simulink model "NPC_threelevel_PI_Controller"  (R2024a)
settings: Solver=ode4  StartTime=0.0  StopTime=0.1  FixedStep=1e-6  MaxStep=1e-4  RelTol=1e-3
InitFcn:
  | v=3000
  | r=0.000001
  | c=1000e-6
  | l=314
  | i=1000
  | r1=1000
  | t=1/3000
  | ma=2
  | f=2*pi*50
  | p1=(2*pi)/3
  | p2=-(2*pi)/3
libraries: spsIGBTDiodeLib x12, spsSeriesRLCBranchLib x12, spsVoltageMeasurementLib x12, simulink x6, spsDiodeLib x6, slpidlib x3, spsRMSLib x3, spsCurrentMeasurementLib x3, spsDCVoltageSourceLib x1, sps_lib x1
settings Model: Creator=dell  LastModifiedBy=prath
settings SolverCC: AlgebraicLoopSolver=TrustRegion
settings DataIOCC: ReturnWorkspaceOutputs=off
settings DebuggingCC: UnconnectedInputMsg=warning  UnconnectedOutputMsg=warning  UnconnectedLineMsg=warning  ArithmeticOperatorsInVariantConditions=warning
settings ModelReferenceCC: EnableRefExpFcnMdlSchedulingChecks=on
settings SFSimCC: SimUseLocalCustomCode=off  CustomCodeUndefinedFunction=UseInterfaceOnly
settings RTWCC: RTWUseLocalCustomCode=off  GPUComputeCapability=3.5
settings CodeAppCC: StateflowObjectComments=on
settings SimscapeCC: SimscapeNormalizeSystem=off

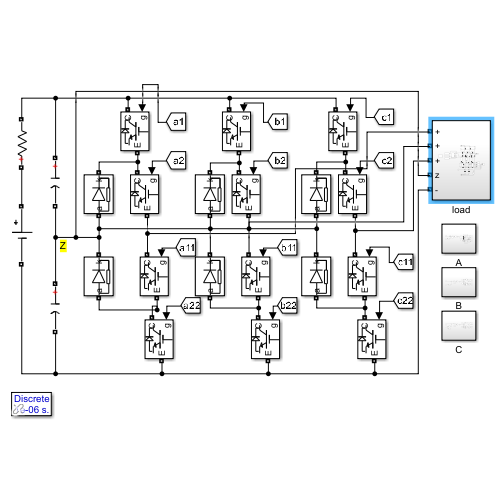
[thumbnail: Simulink's stored preview of the top-level diagram]
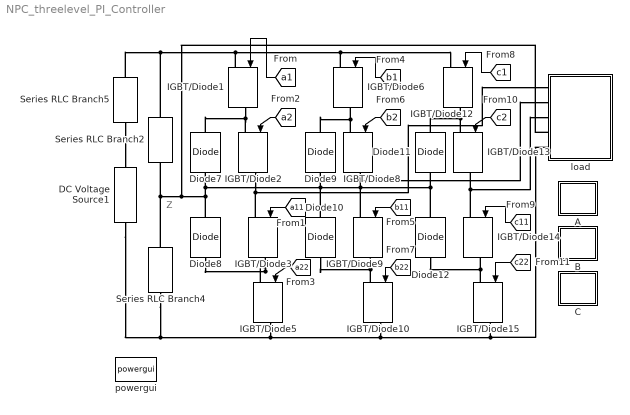
== system NPC_threelevel_PI_Controller ==
  note: Z
  A : Subsystem
  B : Subsystem
  C : Subsystem
  DC Voltage Source1 : spsDCVoltageSourceLib/DC Voltage Source  Amplitude=3000  Measurements=None
  Diode{7..12} (6 alike) : spsDiodeLib/Diode  Ron=0.001  Lon=0  Vf=0.8  IC=0  UseSnubber=0  Rs=500  Cs=250e-9  Measurements=off
  IGBT/Diode{1..3,5..6,8..10,12..15} (12 alike) : spsIGBTDiodeLib/IGBT//Diode  Ron=1e-3  Rs=1e5  Cs=inf  Measurements=off
  Series RLC Branch2 : spsSeriesRLCBranchLib/Series RLC Branch  LConnTagsString=__new0  RConnTagsString=__new0  BranchType=C  Resistance=1  Inductance=1e-3  SetiL0=off  InitialCurrent=0  Capacitance=0.001  Setx0=on  InitialVoltage=1000  Measurements=None
  Series RLC Branch4 : spsSeriesRLCBranchLib/Series RLC Branch  LConnTagsString=__new0  RConnTagsString=__new0  BranchType=C  Resistance=1  Inductance=1e-3  SetiL0=off  InitialCurrent=0  Capacitance=0.001  Setx0=on  InitialVoltage=1000  Measurements=None
  Series RLC Branch5 : spsSeriesRLCBranchLib/Series RLC Branch  LConnTagsString=__new0  RConnTagsString=__new0  BranchType=R  Resistance=r  Inductance=1e-3  SetiL0=off  InitialCurrent=0  Capacitance=1e-6  Setx0=off  InitialVoltage=0  Measurements=None
  load : Subsystem
  powergui : sps_lib/powergui  Priority=1  SimulationMode=Discrete  SampleTime=1e-6  frequency=60  Iterations=50  frequencyindice=0  Pbase=100e6  ErrMax=1e-4  UnitsV=kV  UnitsW=MW  buscounter=0  FunctionMessages=off  echomessages=off  EnableUseOfTLC=off  CurrentSourceSwitches=off  DisableSnubberDevices=off  DisableRonSwitches=off  DisableVfSwitches=off  DisplayEquations=off  AutomaticDiscreteSolvers=off  SolverType=Tustin/Backward Euler (TBE)  Interpol=off  ExternalGateDelay=off  methode=off  Ts=100  x0status=blocks  SPID=on  SwTol=0  HookPort=off  NonlinearTolerance=1e-4  nMaxIteration=100  ContinueOnMaxIteration=off  RestoreLinks=warning  ResistiveCurrentMeasurement=off  Frange=[0:2:500]  Ylog=off  Xlog=on  ShowGrid=off  save=off  variable=ZData  structure=d  ZoomFFT=off  StartTime=0.2  cycles=2  DisplayStyle=1  fundamental=50  FreqAxis=on  MaxFrequency=40000  frequencyindicesteady=1  RmsSteady=1  display=off
  wires:
  [a1] -> IGBT/Diode1/1
  [a2] -> IGBT/Diode2/1
  [a11] -> IGBT/Diode3/1
  [a22] -> IGBT/Diode5/1
  [b1] -> IGBT/Diode6/1
  [b2] -> IGBT/Diode8/1
  [b11] -> IGBT/Diode9/1
  [b22] -> IGBT/Diode10/1
  [c11] -> IGBT/Diode14/1
  [c1] -> IGBT/Diode12/1
  [c2] -> IGBT/Diode13/1
  [c22] -> IGBT/Diode15/1
  connections:
  Diode7/RConn1 -- IGBT/Diode2/LConn1 -- IGBT/Diode1/RConn1
  IGBT/Diode3/LConn1 -- IGBT/Diode2/RConn1 -- load/LConn1
  IGBT/Diode5/LConn1 -- Diode8/LConn1 -- IGBT/Diode3/RConn1
  IGBT/Diode8/LConn1 -- Diode9/RConn1 -- IGBT/Diode6/RConn1
  IGBT/Diode9/LConn1 -- IGBT/Diode8/RConn1 -- load/LConn2
  Diode10/LConn1 -- IGBT/Diode10/LConn1 -- IGBT/Diode9/RConn1
  IGBT/Diode13/LConn1 -- Diode11/RConn1 -- IGBT/Diode12/RConn1
  IGBT/Diode14/LConn1 -- load/LConn3 -- IGBT/Diode13/RConn1
  IGBT/Diode15/LConn1 -- Diode12/LConn1 -- IGBT/Diode14/RConn1
  Series RLC Branch4/LConn1 -- Diode12/RConn1 -- Diode11/LConn1 -- Diode10/RConn1 -- Diode9/LConn1 -- Diode7/LConn1 -- Diode8/RConn1 -- load/LConn4 -- Series RLC Branch2/RConn1
  Series RLC Branch5/LConn1 -- DC Voltage Source1/RConn1
  Series RLC Branch5/RConn1 -- Series RLC Branch2/LConn1 -- IGBT/Diode1/LConn1 -- IGBT/Diode6/LConn1 -- IGBT/Diode12/LConn1
  DC Voltage Source1/LConn1 -- Series RLC Branch4/RConn1 -- IGBT/Diode10/RConn1 -- load/LConn5 -- IGBT/Diode15/RConn1 -- IGBT/Diode5/RConn1

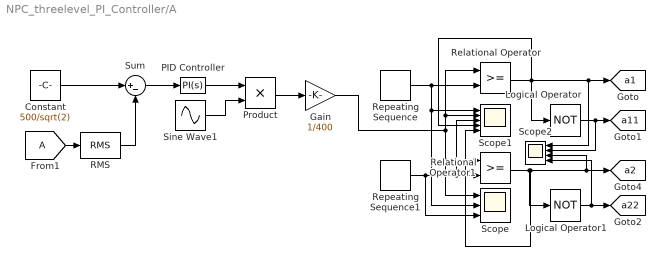
== system NPC_threelevel_PI_Controller/A ==
  Constant : Constant  Value=500/sqrt(2)
  From1 : From  TagVisibility=global
  Gain : Gain  Gain=1/400
  Logical Operator : Logic  Operator=NOT  AllPortsSameDT=off  OutDataTypeStr=boolean
  Logical Operator1 : Logic  Operator=NOT  AllPortsSameDT=off  OutDataTypeStr=boolean
  PID Controller : slpidlib/PID Controller  Controller=PI  Form=Parallel  TimeDomain=Continuous-time  UseExternalTs=off  SampleTime=-1  IntegratorMethod=Forward Euler  FilterMethod=Forward Euler  ControllerParametersSource=internal  P=0.1  I=20  UseKiTs=off  D=0  UseExternalDerivativeSource=off  N=100  UseFilter=on  TunerSelectOption=Transfer Function Based (PID Tuner App)  InitialConditionSource=internal  InitialConditionForIntegrator=0  InitialConditionForFilter=0  DifferentiatorICPrevScaledInput=0  ExternalReset=none  TrackingMode=off  Kt=1  LimitOutput=off  SatLimitsSource=internal  UpperSaturationLimit=inf  LowerSaturationLimit=-inf  LinearizeAsGain=on  AntiWindupMode=none  Kb=1  LimitIntegrator=off  UpperIntegratorSaturationLimit=inf  LowerIntegratorSaturationLimit=-inf  POutMin=[]  POutMax=[]  IOutMin=[]  IOutMax=[]  DOutMin=[]  DOutMax=[]  NOutMin=[]  NOutMax=[]  SumOutMin=[]  SumOutMax=[]  SaturationOutMin=[]  SaturationOutMax=[]  PParamMin=[]  PParamMax=[]  IParamMin=[]  IParamMax=[]  DParamMin=[]  DParamMax=[]  NParamMin=[]  NParamMax=[]  KbParamMin=[]  KbParamMax=[]  KtParamMin=[]  KtParamMax=[]  KbOutMin=[]  KbOutMax=[]  KtOutMin=[]  KtOutMax=[]  IntegratorOutMin=[]  IntegratorOutMax=[]  FilterOutMin=[]  FilterOutMax=[]  SumI1OutMin=[]  SumI1OutMax=[]  SumI2OutMin=[]  SumI2OutMax=[]  SumI3OutMin=[]  SumI3OutMax=[]  SumI4OutMin=[]  SumI4OutMax=[]  SumDOutMin=[]  SumDOutMax=[]  DifferentiatorOutMin=[]  DifferentiatorOutMax=[]  FilterDiffOutCoefMin=[]  FilterDiffOutCoefMax=[]  ReciprocalOutMin=[]  ReciprocalOutMax=[]  SumDenOutMin=[]  SumDenOutMax=[]  SumNumOutMin=[]  SumNumOutMax=[]  DivideOutMin=[]  DivideOutMax=[]  UdiffTsProdOutMin=[]  UdiffTsProdOutMax=[]  NTsProdOutMin=[]  NTsProdOutMax=[]  UintegralTsProdOutMin=[]  UintegralTsProdOutMax=[]  UngainTsProdOutMin=[]  UngainTsProdOutMax=[]  ClampingZeroOutDataTypeStr=Inherit: Inherit via back propagation  ClampingZeroOutMin=[]  ClampingZeroOutMax=[]  FilterDenConstantOutDataTypeStr=Inherit: Inherit via back propagation  FilterDenConstantOutMin=[]  FilterDenConstantOutMax=[]  PCopyOutDataTypeStr=Inherit: Inherit via back propagation  PCopyOutMin=[]  PCopyOutMax=[]  NCopyOutDataTypeStr=Inherit: Inherit via back propagation  NCopyOutMin=[]  NCopyOutMax=[]  IntegratorContinuousStateAttributes=''  IntegratorStateMustResolveToSignalObject=off  IntegratorRTWStateStorageClass=Auto  FilterContinuousStateAttributes=''  FilterStateMustResolveToSignalObject=off  FilterRTWStateStorageClass=Auto  ParallelPVariant=InternalParameters  IdealPVariant=Disabled  IVariant=InternalParameters  DVariant=Disabled  IntegratorVariant=Continuous  SatVariant=Disabled  AWVariant=Passthrough  PCopyVariant=Disabled  TRVariant=Disabled  FdbkBlocksVariant=Forward  IdealPFdbkVariant=Disabled  SatFdbkVariant=Disabled  DerivativeFilterVariant=Disabled  NVariant=Disabled  NCopyVariant=Disabled_SignalSpec  FilterICVariant=Disabled  IntegratorICVariant=InternalICs  ExternalResetVariant=Disabled  TRSumVariant=Passthrough  SumFdbkVariant=Disabled  SumVariant=Sum_PI  TsampFilterVariant=InternalTs  TsampNgainVariant=Passthrough  TsampIntegralVariant=Disabled_SignalSpec  ExternalSaturationOutDataTypeStr=Inherit: Same as second input  DerivativeSourceVariant=Disabled
  Product : Product
  RMS : spsRMSLib/RMS  TrueRMS=on  Freq=50  RMSInit=230  Ts=0
  Relational Operator : RelationalOperator  OutDataTypeStr=boolean  RndMeth=Simplest  InputSameDT=off
  Relational Operator1 : RelationalOperator  OutDataTypeStr=boolean  RndMeth=Simplest  InputSameDT=off
  Repeating Sequence : simulink/Sources/Repeating Sequence  rep_seq_t=[0 0.00005 0.0001]  rep_seq_y=[0 1 0]
  Repeating Sequence1 : simulink/Sources/Repeating Sequence  rep_seq_t=[0 0.00005 0.0001]  rep_seq_y=[-1 0 -1]
  Scope : Scope  NumInputPorts=3
  Scope1 : Scope  NumInputPorts=5
  Scope2 : Scope  NumInputPorts=4
  Sine Wave1 : Sin  Frequency=2*pi*50  SampleTime=0
  Sum : Sum  Inputs=|+-
  tag scope: a11=global, a1=global, a22=global, a2=global
  wires:
  Logical Operator/1 -> Scope2/2, [a11]
  Logical Operator1/1 -> [a22], Scope2/4
  Repeating Sequence/1 -> Scope/2, Scope1/1, Relational Operator/2
  Repeating Sequence1/1 -> Scope/3, Scope1/3, Relational Operator1/2
  Relational Operator/1 -> Scope1/4, Logical Operator/1, Scope2/1, [a1]
  Relational Operator1/1 -> Logical Operator1/1, Scope1/5, Scope2/3, [a2]
  Gain/1 -> Scope/1, Relational Operator1/1, Scope1/2, Relational Operator/1
  Constant/1 -> Sum/1
  From1/1 -> RMS/1
  RMS/1 -> Sum/2
  PID Controller/1 -> Product/1
  Sine Wave1/1 -> Product/2
  Product/1 -> Gain/1
  Sum/1 -> PID Controller/1

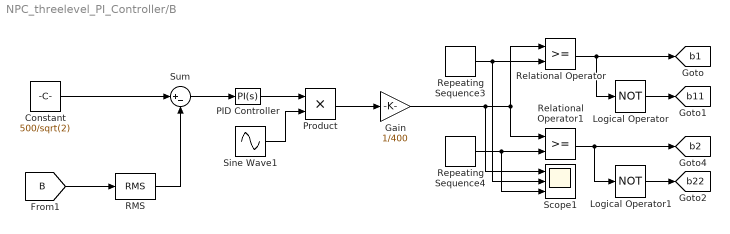
== system NPC_threelevel_PI_Controller/B ==
  Constant : Constant  Value=500/sqrt(2)
  Gain : Gain  Gain=1/400
  Logical Operator : Logic  Operator=NOT  AllPortsSameDT=off  OutDataTypeStr=boolean
  Logical Operator1 : Logic  Operator=NOT  AllPortsSameDT=off  OutDataTypeStr=boolean
  PID Controller : slpidlib/PID Controller  Controller=PI  Form=Parallel  TimeDomain=Continuous-time  UseExternalTs=off  SampleTime=-1  IntegratorMethod=Forward Euler  FilterMethod=Forward Euler  ControllerParametersSource=internal  P=0.1  I=20  UseKiTs=off  D=0  UseExternalDerivativeSource=off  N=100  UseFilter=on  TunerSelectOption=Transfer Function Based (PID Tuner App)  InitialConditionSource=internal  InitialConditionForIntegrator=0  InitialConditionForFilter=0  DifferentiatorICPrevScaledInput=0  ExternalReset=none  TrackingMode=off  Kt=1  LimitOutput=off  SatLimitsSource=internal  UpperSaturationLimit=inf  LowerSaturationLimit=-inf  LinearizeAsGain=on  AntiWindupMode=none  Kb=1  LimitIntegrator=off  UpperIntegratorSaturationLimit=inf  LowerIntegratorSaturationLimit=-inf  POutMin=[]  POutMax=[]  IOutMin=[]  IOutMax=[]  DOutMin=[]  DOutMax=[]  NOutMin=[]  NOutMax=[]  SumOutMin=[]  SumOutMax=[]  SaturationOutMin=[]  SaturationOutMax=[]  PParamMin=[]  PParamMax=[]  IParamMin=[]  IParamMax=[]  DParamMin=[]  DParamMax=[]  NParamMin=[]  NParamMax=[]  KbParamMin=[]  KbParamMax=[]  KtParamMin=[]  KtParamMax=[]  KbOutMin=[]  KbOutMax=[]  KtOutMin=[]  KtOutMax=[]  IntegratorOutMin=[]  IntegratorOutMax=[]  FilterOutMin=[]  FilterOutMax=[]  SumI1OutMin=[]  SumI1OutMax=[]  SumI2OutMin=[]  SumI2OutMax=[]  SumI3OutMin=[]  SumI3OutMax=[]  SumI4OutMin=[]  SumI4OutMax=[]  SumDOutMin=[]  SumDOutMax=[]  DifferentiatorOutMin=[]  DifferentiatorOutMax=[]  FilterDiffOutCoefMin=[]  FilterDiffOutCoefMax=[]  ReciprocalOutMin=[]  ReciprocalOutMax=[]  SumDenOutMin=[]  SumDenOutMax=[]  SumNumOutMin=[]  SumNumOutMax=[]  DivideOutMin=[]  DivideOutMax=[]  UdiffTsProdOutMin=[]  UdiffTsProdOutMax=[]  NTsProdOutMin=[]  NTsProdOutMax=[]  UintegralTsProdOutMin=[]  UintegralTsProdOutMax=[]  UngainTsProdOutMin=[]  UngainTsProdOutMax=[]  ClampingZeroOutDataTypeStr=Inherit: Inherit via back propagation  ClampingZeroOutMin=[]  ClampingZeroOutMax=[]  FilterDenConstantOutDataTypeStr=Inherit: Inherit via back propagation  FilterDenConstantOutMin=[]  FilterDenConstantOutMax=[]  PCopyOutDataTypeStr=Inherit: Inherit via back propagation  PCopyOutMin=[]  PCopyOutMax=[]  NCopyOutDataTypeStr=Inherit: Inherit via back propagation  NCopyOutMin=[]  NCopyOutMax=[]  IntegratorContinuousStateAttributes=''  IntegratorStateMustResolveToSignalObject=off  IntegratorRTWStateStorageClass=Auto  FilterContinuousStateAttributes=''  FilterStateMustResolveToSignalObject=off  FilterRTWStateStorageClass=Auto  ParallelPVariant=InternalParameters  IdealPVariant=Disabled  IVariant=InternalParameters  DVariant=Disabled  IntegratorVariant=Continuous  SatVariant=Disabled  AWVariant=Passthrough  PCopyVariant=Disabled  TRVariant=Disabled  FdbkBlocksVariant=Forward  IdealPFdbkVariant=Disabled  SatFdbkVariant=Disabled  DerivativeFilterVariant=Disabled  NVariant=Disabled  NCopyVariant=Disabled_SignalSpec  FilterICVariant=Disabled  IntegratorICVariant=InternalICs  ExternalResetVariant=Disabled  TRSumVariant=Passthrough  SumFdbkVariant=Disabled  SumVariant=Sum_PI  TsampFilterVariant=InternalTs  TsampNgainVariant=Passthrough  TsampIntegralVariant=Disabled_SignalSpec  ExternalSaturationOutDataTypeStr=Inherit: Same as second input  DerivativeSourceVariant=Disabled
  Product : Product
  RMS : spsRMSLib/RMS  TrueRMS=on  Freq=50  RMSInit=230  Ts=0
  Relational Operator : RelationalOperator  OutDataTypeStr=boolean  RndMeth=Simplest  InputSameDT=off
  Relational Operator1 : RelationalOperator  OutDataTypeStr=boolean  RndMeth=Simplest  InputSameDT=off
  Repeating Sequence3 : simulink/Sources/Repeating Sequence  rep_seq_t=[0 0.00005 0.0001]  rep_seq_y=[0 1 0]
  Repeating Sequence4 : simulink/Sources/Repeating Sequence  rep_seq_t=[0 0.00005 0.0001]  rep_seq_y=[-1 0 -1]
  Scope1 : Scope  NumInputPorts=3
  Sine Wave1 : Sin  Frequency=2*pi*50  Phase=p2  SampleTime=0
  Sum : Sum  Inputs=|+-
  tag scope: b11=global, b1=global, b22=global, b2=global
  wires:
  Logical Operator1/1 -> [b22]
  Repeating Sequence3/1 -> Scope1/2, Relational Operator/2
  Repeating Sequence4/1 -> Scope1/3, Relational Operator1/2
  Gain/1 -> Scope1/1, Relational Operator1/1, Relational Operator/1
  Relational Operator1/1 -> Logical Operator1/1, [b2]
  Relational Operator/1 -> Logical Operator/1, [b1]
  Logical Operator/1 -> [b11]
  Product/1 -> Gain/1
  Constant/1 -> Sum/1
  [B] -> RMS/1
  RMS/1 -> Sum/2
  Sum/1 -> PID Controller/1
  PID Controller/1 -> Product/1
  Sine Wave1/1 -> Product/2

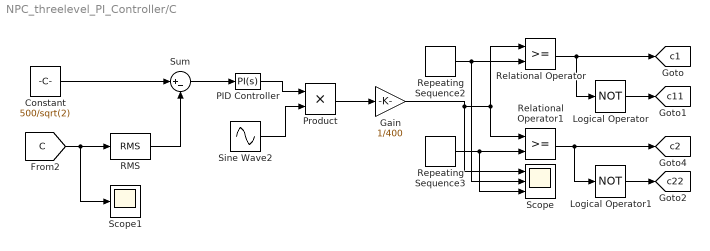
== system NPC_threelevel_PI_Controller/C ==
  Constant : Constant  Value=500/sqrt(2)
  Gain : Gain  Gain=1/400
  Logical Operator : Logic  Operator=NOT  AllPortsSameDT=off  OutDataTypeStr=boolean
  Logical Operator1 : Logic  Operator=NOT  AllPortsSameDT=off  OutDataTypeStr=boolean
  PID Controller : slpidlib/PID Controller  Controller=PI  Form=Parallel  TimeDomain=Continuous-time  UseExternalTs=off  SampleTime=-1  IntegratorMethod=Forward Euler  FilterMethod=Forward Euler  ControllerParametersSource=internal  P=0.1  I=20  UseKiTs=off  D=0  UseExternalDerivativeSource=off  N=100  UseFilter=on  TunerSelectOption=Transfer Function Based (PID Tuner App)  InitialConditionSource=internal  InitialConditionForIntegrator=0  InitialConditionForFilter=0  DifferentiatorICPrevScaledInput=0  ExternalReset=none  TrackingMode=off  Kt=1  LimitOutput=off  SatLimitsSource=internal  UpperSaturationLimit=inf  LowerSaturationLimit=-inf  LinearizeAsGain=on  AntiWindupMode=none  Kb=1  LimitIntegrator=off  UpperIntegratorSaturationLimit=inf  LowerIntegratorSaturationLimit=-inf  POutMin=[]  POutMax=[]  IOutMin=[]  IOutMax=[]  DOutMin=[]  DOutMax=[]  NOutMin=[]  NOutMax=[]  SumOutMin=[]  SumOutMax=[]  SaturationOutMin=[]  SaturationOutMax=[]  PParamMin=[]  PParamMax=[]  IParamMin=[]  IParamMax=[]  DParamMin=[]  DParamMax=[]  NParamMin=[]  NParamMax=[]  KbParamMin=[]  KbParamMax=[]  KtParamMin=[]  KtParamMax=[]  KbOutMin=[]  KbOutMax=[]  KtOutMin=[]  KtOutMax=[]  IntegratorOutMin=[]  IntegratorOutMax=[]  FilterOutMin=[]  FilterOutMax=[]  SumI1OutMin=[]  SumI1OutMax=[]  SumI2OutMin=[]  SumI2OutMax=[]  SumI3OutMin=[]  SumI3OutMax=[]  SumI4OutMin=[]  SumI4OutMax=[]  SumDOutMin=[]  SumDOutMax=[]  DifferentiatorOutMin=[]  DifferentiatorOutMax=[]  FilterDiffOutCoefMin=[]  FilterDiffOutCoefMax=[]  ReciprocalOutMin=[]  ReciprocalOutMax=[]  SumDenOutMin=[]  SumDenOutMax=[]  SumNumOutMin=[]  SumNumOutMax=[]  DivideOutMin=[]  DivideOutMax=[]  UdiffTsProdOutMin=[]  UdiffTsProdOutMax=[]  NTsProdOutMin=[]  NTsProdOutMax=[]  UintegralTsProdOutMin=[]  UintegralTsProdOutMax=[]  UngainTsProdOutMin=[]  UngainTsProdOutMax=[]  ClampingZeroOutDataTypeStr=Inherit: Inherit via back propagation  ClampingZeroOutMin=[]  ClampingZeroOutMax=[]  FilterDenConstantOutDataTypeStr=Inherit: Inherit via back propagation  FilterDenConstantOutMin=[]  FilterDenConstantOutMax=[]  PCopyOutDataTypeStr=Inherit: Inherit via back propagation  PCopyOutMin=[]  PCopyOutMax=[]  NCopyOutDataTypeStr=Inherit: Inherit via back propagation  NCopyOutMin=[]  NCopyOutMax=[]  IntegratorContinuousStateAttributes=''  IntegratorStateMustResolveToSignalObject=off  IntegratorRTWStateStorageClass=Auto  FilterContinuousStateAttributes=''  FilterStateMustResolveToSignalObject=off  FilterRTWStateStorageClass=Auto  ParallelPVariant=InternalParameters  IdealPVariant=Disabled  IVariant=InternalParameters  DVariant=Disabled  IntegratorVariant=Continuous  SatVariant=Disabled  AWVariant=Passthrough  PCopyVariant=Disabled  TRVariant=Disabled  FdbkBlocksVariant=Forward  IdealPFdbkVariant=Disabled  SatFdbkVariant=Disabled  DerivativeFilterVariant=Disabled  NVariant=Disabled  NCopyVariant=Disabled_SignalSpec  FilterICVariant=Disabled  IntegratorICVariant=InternalICs  ExternalResetVariant=Disabled  TRSumVariant=Passthrough  SumFdbkVariant=Disabled  SumVariant=Sum_PI  TsampFilterVariant=InternalTs  TsampNgainVariant=Passthrough  TsampIntegralVariant=Disabled_SignalSpec  ExternalSaturationOutDataTypeStr=Inherit: Same as second input  DerivativeSourceVariant=Disabled
  Product : Product
  RMS : spsRMSLib/RMS  TrueRMS=on  Freq=50  RMSInit=230  Ts=0
  Relational Operator : RelationalOperator  OutDataTypeStr=boolean  RndMeth=Simplest  InputSameDT=off
  Relational Operator1 : RelationalOperator  OutDataTypeStr=boolean  RndMeth=Simplest  InputSameDT=off
  Repeating Sequence2 : simulink/Sources/Repeating Sequence  rep_seq_t=[0 0.00005 0.0001]  rep_seq_y=[0 1 0]
  Repeating Sequence3 : simulink/Sources/Repeating Sequence  rep_seq_t=[0 0.00005 0.0001]  rep_seq_y=[-1 0 -1]
  Scope : Scope  NumInputPorts=3
  Scope1 : Scope
  Sine Wave2 : Sin  Frequency=2*pi*50  Phase=p1  SampleTime=0
  Sum : Sum  Inputs=|+-
  tag scope: c11=global, c1=global, c22=global, c2=global
  wires:
  Logical Operator1/1 -> [c22]
  Repeating Sequence2/1 -> Scope/2, Relational Operator/2
  Repeating Sequence3/1 -> Scope/3, Relational Operator1/2
  Gain/1 -> Scope/1, Relational Operator1/1, Relational Operator/1
  Relational Operator1/1 -> Logical Operator1/1, [c2]
  Relational Operator/1 -> Logical Operator/1, [c1]
  Logical Operator/1 -> [c11]
  Constant/1 -> Sum/1
  [C] -> Scope1/1, RMS/1
  RMS/1 -> Sum/2
  Sum/1 -> PID Controller/1
  PID Controller/1 -> Product/1
  Sine Wave2/1 -> Product/2
  Product/1 -> Gain/1

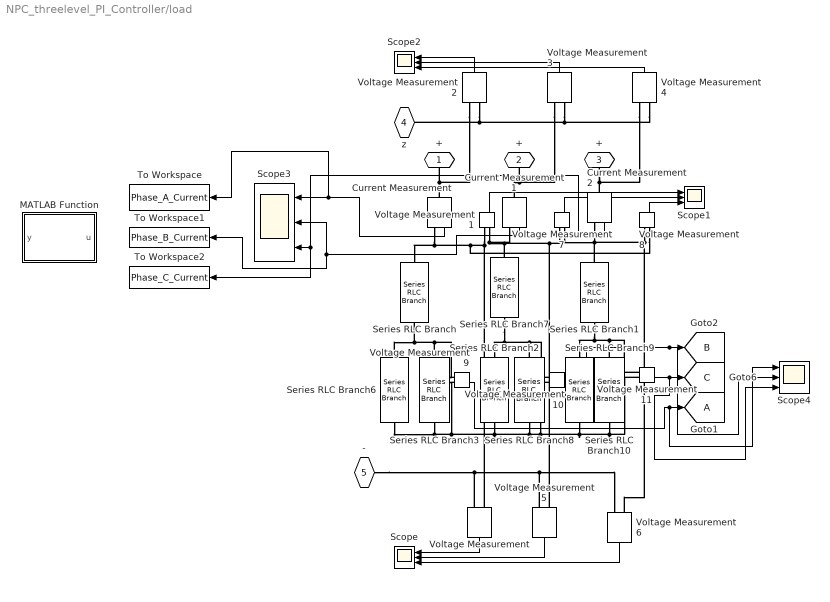
== system NPC_threelevel_PI_Controller/load ==
  Current Measurement : spsCurrentMeasurementLib/Current Measurement  PhasorSimulation=off  OutputType=Complex  PSBequivalent=0
  Current Measurement1 : spsCurrentMeasurementLib/Current Measurement  PhasorSimulation=off  OutputType=Complex  PSBequivalent=0
  Current Measurement2 : spsCurrentMeasurementLib/Current Measurement  PhasorSimulation=off  OutputType=Complex  PSBequivalent=0
  Goto1 : Goto  TagVisibility=global
  MATLAB Function : MATLAB Function  TreatAsAtomicUnit=on
  Scope{,1..4} (5 alike) : Scope  NumInputPorts=3
  Series RLC Branch : spsSeriesRLCBranchLib/Series RLC Branch  LConnTagsString=__new0  RConnTagsString=__new0  BranchType=RL  Resistance=0.002  Inductance=4e-2  SetiL0=off  InitialCurrent=0  Capacitance=1e-3  Setx0=off  InitialVoltage=0  Measurements=None
  Series RLC Branch1 : spsSeriesRLCBranchLib/Series RLC Branch  LConnTagsString=__new0  RConnTagsString=__new0  BranchType=RL  Resistance=0.002  Inductance=4e-2  SetiL0=off  InitialCurrent=0  Capacitance=1e-3  Setx0=off  InitialVoltage=0  Measurements=None
  Series RLC Branch10 : spsSeriesRLCBranchLib/Series RLC Branch  LConnTagsString=__new0  RConnTagsString=__new0  BranchType=RC  Resistance=0.002  Inductance=4e-3  SetiL0=off  InitialCurrent=0  Capacitance=6e-6  Setx0=off  InitialVoltage=0  Measurements=None
  Series RLC Branch2 : spsSeriesRLCBranchLib/Series RLC Branch  LConnTagsString=__new0  RConnTagsString=__new0  BranchType=R  Resistance=20  Inductance=4e-3  SetiL0=off  InitialCurrent=0  Capacitance=6e-6  Setx0=off  InitialVoltage=0  Measurements=None
  Series RLC Branch3 : spsSeriesRLCBranchLib/Series RLC Branch  LConnTagsString=__new0  RConnTagsString=__new0  BranchType=RC  Resistance=0.002  Inductance=4e-3  SetiL0=off  InitialCurrent=0  Capacitance=6e-6  Setx0=off  InitialVoltage=0  Measurements=None
  Series RLC Branch6 : spsSeriesRLCBranchLib/Series RLC Branch  LConnTagsString=__new0  RConnTagsString=__new0  BranchType=R  Resistance=20  Inductance=4e-3  SetiL0=off  InitialCurrent=0  Capacitance=6e-6  Setx0=off  InitialVoltage=0  Measurements=None
  Series RLC Branch7 : spsSeriesRLCBranchLib/Series RLC Branch  LConnTagsString=__new0  RConnTagsString=__new0  BranchType=RL  Resistance=0.002  Inductance=4e-2  SetiL0=off  InitialCurrent=0  Capacitance=1e-3  Setx0=off  InitialVoltage=0  Measurements=None
  Series RLC Branch8 : spsSeriesRLCBranchLib/Series RLC Branch  LConnTagsString=__new0  RConnTagsString=__new0  BranchType=RC  Resistance=0.002  Inductance=4e-3  SetiL0=off  InitialCurrent=0  Capacitance=6e-6  Setx0=off  InitialVoltage=0  Measurements=None
  Series RLC Branch9 : spsSeriesRLCBranchLib/Series RLC Branch  LConnTagsString=__new0  RConnTagsString=__new0  BranchType=R  Resistance=20  Inductance=4e-3  SetiL0=off  InitialCurrent=0  Capacitance=6e-6  Setx0=off  InitialVoltage=0  Measurements=None
  To Workspace : ToWorkspace  VariableName=Phase_A_Current  SampleTime=0.0002
  To Workspace1 : ToWorkspace  VariableName=Phase_B_Current  SampleTime=0.0002
  To Workspace2 : ToWorkspace  VariableName=Phase_C_Current  SampleTime=0.0002
  Voltage Measurement{,1..11} (12 alike) : spsVoltageMeasurementLib/Voltage Measurement  PhasorSimulation=off  OutputType=Complex  PSBequivalent=0
  + : PMIOPort  Side=Left
  "+  " : PMIOPort  Port=2  Side=Left
  "+   " : PMIOPort  Port=3  Side=Left
  z : PMIOPort  Port=4  Side=Left
  - : PMIOPort  Port=5  Side=Left
  tag scope: B=global, C=global
  wires:
  Current Measurement/1 -> To Workspace/1, Scope3/1
  Voltage Measurement/1 -> Scope/1
  Voltage Measurement5/1 -> Scope/2
  Voltage Measurement6/1 -> Scope/3
  Voltage Measurement1/1 -> Scope1/1
  Voltage Measurement7/1 -> Scope1/2
  Voltage Measurement8/1 -> Scope1/3
  Voltage Measurement2/1 -> Scope2/1
  Voltage Measurement3/1 -> Scope2/2
  Voltage Measurement4/1 -> Scope2/3
  Current Measurement1/1 -> Scope3/2, To Workspace1/1
  Current Measurement2/1 -> To Workspace2/1, Scope3/3
  Voltage Measurement9/1 -> Scope4/1, Goto1/1
  Voltage Measurement10/1 -> Scope4/2, [B]
  Voltage Measurement11/1 -> Scope4/3, [C]
  connections:
  Voltage Measurement7/LConn2 -- Voltage Measurement8/LConn1 -- Voltage Measurement6/LConn1 -- Series RLC Branch1/LConn1 -- Current Measurement2/RConn1
  "+  "/RConn1 -- Current Measurement1/LConn1 -- Voltage Measurement3/LConn1
  Series RLC Branch6/RConn1 -- Voltage Measurement9/LConn2 -- Voltage Measurement10/LConn2 -- Voltage Measurement11/LConn2 -- Series RLC Branch10/RConn1 -- Series RLC Branch9/RConn1 -- Series RLC Branch8/RConn1 -- Series RLC Branch2/RConn1 -- Series RLC Branch3/RConn1
  Current Measurement/RConn1 -- Voltage Measurement8/LConn2 -- Voltage Measurement/LConn1 -- Voltage Measurement1/LConn1 -- Series RLC Branch/LConn1
  +/RConn1 -- Current Measurement/LConn1 -- Voltage Measurement2/LConn1
  Voltage Measurement2/LConn2 -- Voltage Measurement4/LConn2 -- Voltage Measurement3/LConn2 -- z/RConn1
  -/RConn1 -- Voltage Measurement/LConn2 -- Voltage Measurement6/LConn2 -- Voltage Measurement5/LConn2
  Voltage Measurement7/LConn1 -- Series RLC Branch7/LConn1 -- Current Measurement1/RConn1 -- Voltage Measurement1/LConn2 -- Voltage Measurement5/LConn1
  Voltage Measurement4/LConn1 -- Current Measurement2/LConn1 -- "+   "/RConn1
  Series RLC Branch3/LConn1 -- Voltage Measurement9/LConn1 -- Series RLC Branch6/LConn1 -- Series RLC Branch/RConn1
  Series RLC Branch7/RConn1 -- Voltage Measurement10/LConn1 -- Series RLC Branch8/LConn1 -- Series RLC Branch2/LConn1
  Series RLC Branch1/RConn1 -- Voltage Measurement11/LConn1 -- Series RLC Branch10/LConn1 -- Series RLC Branch9/LConn1

== matlab function NPC_threelevel_PI_Controller/load/MATLAB Function ==
  data: u input; y output
function y = fcn(u)

y = u;
